simulink model "Drone_Model"  (R2019b)
settings: Solver=VariableStepAuto  StartTime=0.0  StopTime=6  RelTol=1e-3
values from neighbouring files (symbols this model uses):
  A = double(round(subs(J_x,   [states, inputs], [trim_state, trim_input])*1000)/1000)    [state_decoupling.m]
  Aaileron = A(5:8,5:8)    [state_decoupling.m]
  Aelevator = A(1:4,1:4)    [state_decoupling.m]
  Arudder = A(11:12,11:12)    [state_decoupling.m]
  Athrust = A(9:10,9:10)    [state_decoupling.m]
  B = B*MotorMix    [state_decoupling.m]
  Baileron = B(5:8,3)    [state_decoupling.m]
  Belevator = B(1:4,2)    [state_decoupling.m]
  Brudder = B(11:12,4)    [state_decoupling.m]
  Bthrust = B(9:10,1)    [state_decoupling.m]
  C = double(round(subs(J_y,   [states, inputs], [trim_state, trim_input])*1000)/1000)    [state_decoupling.m]
  C_P = 0.041    [state_decoupling.m]
  C_rollpitch = rho*prop_dia^4*prop_dist/sqrt(2)*[                 1  -1  -1   1 ;                 1   1  -1  -1 ;                 0   0   0   0 ; ]    [state_decoupling.m]
  C_T = [0.069075;4.95e-05]    [state_decoupling.m]
  C_yaw = rho*prop_dia^5/(2*pi)*[                 0   0   0   0 ;                 0   0   0   0 ;                -1   1  -1   1 ; ]    [state_decoupling.m]
  Caileron = [0 1 0 0; 0 0 0 1; 0 0 0 0]    [state_decoupling.m]
  Celevator = [0 1 0 0; 0 0 0 1; 0 0 0 0]    [state_decoupling.m]
  Crudder = [0 1]    [state_decoupling.m]
  Cthrust = [ 1 0; -1 0; 0 0]    [state_decoupling.m]
  D = D*MotorMix    [state_decoupling.m]
  Daileron = [0 ; 0 ; 0]    [state_decoupling.m]
  Delevator = [0 ; 0 ; 0]    [state_decoupling.m]
  Drudder = 0    [state_decoupling.m]
  Dthrust = [0 ; 0 ; D(4,1)]    [state_decoupling.m]
  g = [0;0;UAV_mass*9.81]    [state_decoupling.m]
  J = [      Jxx   0   0 ;       0   Jyy  0 ;       0    0  Jzz; ]    [state_decoupling.m]
  Jinv = inv(J)    [state_decoupling.m]
  MotorMix = [                 1  1  1 -1 ;                 1  1 -1  1 ;                 1 -1 -1 -1 ;                 1 -1  1  1 ; ]    [state_decoupling.m]
  Prop_H = 2*pi*Jprop*[               0  0  0  0 ;               0  0  0  0 ;               1 -1  1 -1 ; ]    [state_decoupling.m]
  Thrust_Sum = rho*prop_dia^4*[                 0   0   0   0 ;                 0   0   0   0 ;                -1  -1  -1  -1 ; ]    [state_decoupling.m]
  trim_input = [293,293,293,293]    [state_decoupling.m]
  trim_state = [0,0,0,0,0,0,0,0,0,0,0,0]    [state_decoupling.m]
  UAV_mass = 0.068    [state_decoupling.m]
undefined symbols (not defined in the file or in its folder): TEAR
libraries: simulink x8, vrlib x3, dspmtrx3 x1
settings Model: Creator=crbon  LastModifiedBy=Chris

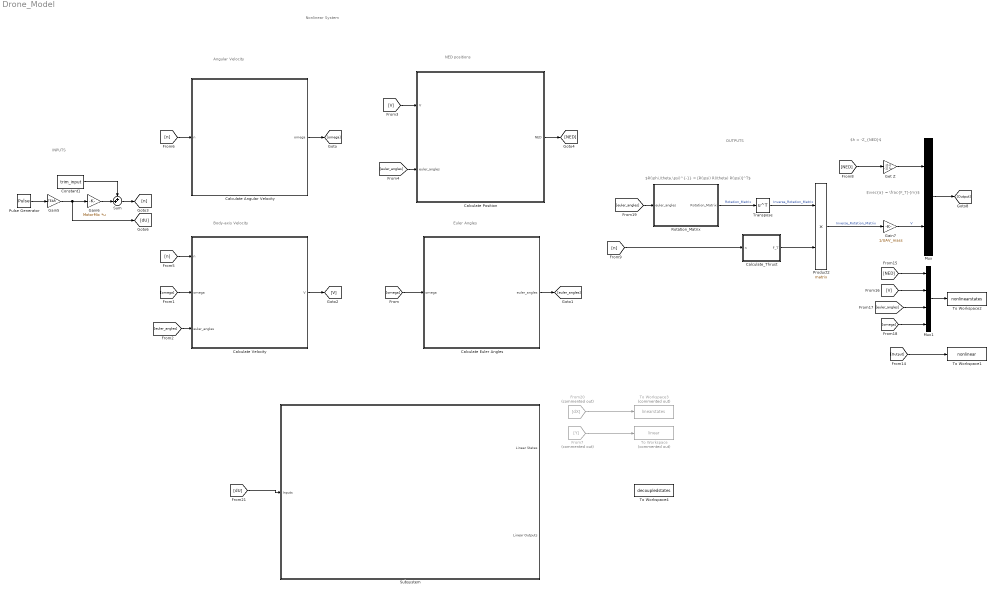
== system Drone_Model ==
  note: Nonlinear System
  note: Euler Angles
  note: NED positions
  note: $\vec{a} = \frac{F_T}{m}$
  note: $h = -Z_{NED}$
  note: $R(\phi,\theta,\psi)^{-1} = [R(\psi) R(\theta) R(\psi)]^T$
  note: OUTPUTS
  note: INPUTS
  note: Angular Velocity
  note: Body-axis Velocity
  Calculate Angular Velocity : Subsystem
  Calculate Euler Angles : Subsystem
  Calculate Position : Subsystem
  Calculate Velocity : Subsystem
  Calculate_Thrust : Subsystem
  Constant1 : Constant  Value=trim_input
  From20 : From  Commented=on  GotoTag=dX
  From7 : From  Commented=on  GotoTag=Y
  Gain5 : Gain  Gain=TEAR
      settings: AttributesFormatString=%<Gain>
  Gain6 : Gain  Gain=MotorMix  Multiplication=Matrix(K*u)
      settings: AttributesFormatString=%<Gain>
  Gain7 : Gain  Gain=1/UAV_mass
      settings: AttributesFormatString=%<Gain>
  Get Z : Gain  Gain=[0 0 -1]  Multiplication=Matrix(K*u)
  Mux : Mux  Inputs=2
  Mux1 : Mux
  Product2 : Product  Multiplication=Matrix(*)
  Pulse Generator : DiscretePulseGenerator  PulseType=Time based  Amplitude=0.05  Period=10  PulseWidth=40  PhaseDelay=1
  Rotation_Matrix : Subsystem
  Subsystem : Subsystem
  Sum : Sum  Inputs=++|
  To Workspace : ToWorkspace  Commented=on  VariableName=linear  SaveFormat=Timeseries  SampleTime=-1
  To Workspace1 : ToWorkspace  VariableName=nonlinear  SaveFormat=Timeseries  SampleTime=-1
  To Workspace2 : ToWorkspace  VariableName=nonlinearstates  SaveFormat=Timeseries  SampleTime=-1
  To Workspace3 : ToWorkspace  Commented=on  VariableName=linearstates  SaveFormat=Timeseries  SampleTime=-1
  To Workspace4 : ToWorkspace  VariableName=decoupledstates  SaveFormat=Timeseries  SampleTime=-1
  Transpose : Math  Operator=transpose  SignedPower=off  SaturateOnIntegerOverflow=on
  wires:
  [omega] -> Calculate Euler Angles/1(omega)
  Calculate Angular Velocity/1(omega) -> [omega]
  [omega] -> Calculate Velocity/2(omega)
  Calculate Euler Angles/1(euler_angles) -> [euler_angles]
  [euler_angles] -> Calculate Velocity/3(euler_angles)
  Calculate Velocity/1(V) -> [V]
  [V] -> Calculate Position/1("V ")
  [euler_angles] -> Calculate Position/2(euler_angles)
  [n] -> Calculate Velocity/1(n)
  [n] -> Calculate Angular Velocity/1(n)
  Calculate Position/1(NED) -> [NED]
  [NED] -> Get Z/1
  Get Z/1 -> Mux/1
  [n] -> Calculate_Thrust/1(n)
  Calculate_Thrust/1(F_T) -> Product2/2
  Gain7/1 -> Mux/2  "V"
  Mux/1 -> [Output]
  From7/1 -> To Workspace/1
  [Output] -> To Workspace1/1
  Constant1/1 -> Sum/1
  [NED] -> Mux1/1
  [V] -> Mux1/2
  [euler_angles] -> Mux1/3
  [omega] -> Mux1/4
  Mux1/1 -> To Workspace2/1
  Pulse Generator/1 -> Gain5/1
  Product2/1 -> Gain7/1  "Inverse_Rotation_Matrix"
  Rotation_Matrix/1(Rotation_Matrix) -> Transpose/1  "Rotation_Matrix"
  [euler_angles] -> Rotation_Matrix/1("euler_angles ")
  Transpose/1 -> Product2/1  "Inverse_Rotation_Matrix"
  From20/1 -> To Workspace3/1
  Gain5/1 -> Gain6/1, [dU]
  Sum/1 -> [n]
  Gain6/1 -> Sum/2
  [dU] -> Subsystem/1("Inputs ")

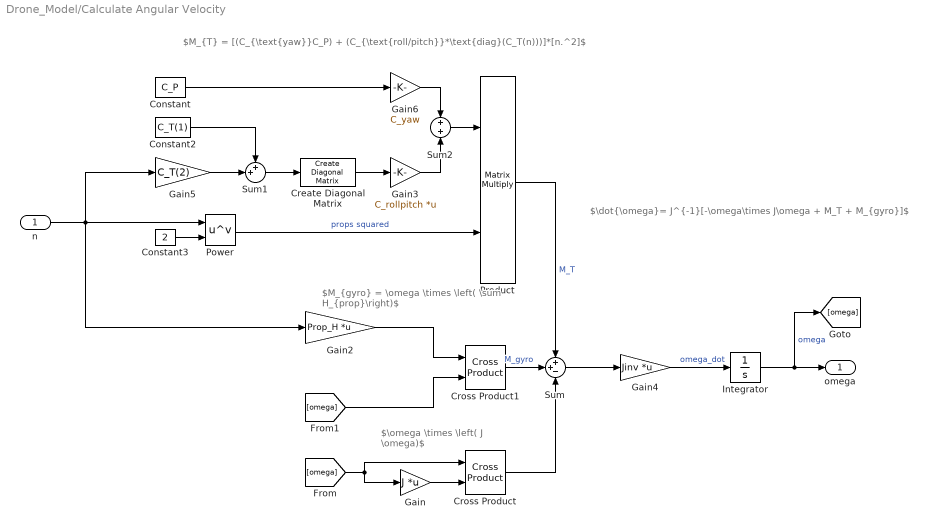
== system Drone_Model/Calculate Angular Velocity ==
  note: $M_{gyro} = \omega \times \left( \sum H_{prop}\right)$
  note: $\dot{\omega}= J^{-1}[-\omega\times J\omega + M_T + M_{gyro}]$
  note: $\omega \times \left( J \omega)$
  note: $M_{T} = [(C_{\text{yaw}}C_P) + (C_{\text{roll/pitch}}*\text{diag}(C_T(n)))]*[n.^2]$
  n : Inport
  Constant : Constant  Value=C_P
  Constant2 : Constant  Value=C_T(1)
  Constant3 : Constant  Value=2
  Create Diagonal Matrix : dspmtrx3/Create Diagonal Matrix
      settings: SourceProductName=DSP System Toolbox  SourceProductBaseCode=DS
  Cross Product : vrlib/Utilities/Cross Product
      settings: SourceProductName=Simulink
  Cross Product1 : vrlib/Utilities/Cross Product
      settings: SourceProductName=Simulink
  Gain : Gain  Gain=J  Multiplication=Matrix(K*u)
  Gain2 : Gain  Gain=Prop_H  Multiplication=Matrix(K*u)
  Gain3 : Gain  Gain=C_rollpitch  Multiplication=Matrix(K*u)
      settings: AttributesFormatString=%<Gain>
  Gain4 : Gain  Gain=Jinv  Multiplication=Matrix(K*u)
      settings: AttributesFormatString=%<Gain>
  Gain5 : Gain  Gain=C_T(2)
  Gain6 : Gain  Gain=C_yaw
      settings: AttributesFormatString=%<Gain>
  Integrator : Integrator  InitialCondition=[0;0;0]
  Power : Math  Operator=pow  SignedPower=off  SaturateOnIntegerOverflow=on
  Product : Product  Multiplication=Matrix(*)
  Sum : Sum  Inputs=++-
  Sum1 : Sum  Inputs=++|
  Sum2 : Sum  Inputs=+|+
  omega : Outport
  wires:
  Sum/1 -> Gain4/1
  [omega] -> Gain/1, Cross Product/1
  Cross Product/1 -> Sum/3
  [omega] -> Cross Product1/2
  Gain2/1 -> Cross Product1/1
  Cross Product1/1 -> Sum/2  "M_gyro"
  Gain4/1 -> Integrator/1  "omega_dot"
  Gain/1 -> Cross Product/2
  Integrator/1 -> [omega], omega/1  "omega"
  Product/1 -> Sum/1  "M_T"
  Create Diagonal Matrix/1 -> Gain3/1
  Sum2/1 -> Product/1
  Sum1/1 -> Create Diagonal Matrix/1
  Constant/1 -> Gain6/1
  Power/1 -> Product/2  "props squared"
  Gain6/1 -> Sum2/1
  Gain5/1 -> Sum1/2
  Gain3/1 -> Sum2/2
  n/1 -> Gain2/1, Power/1, Gain5/1
  Constant2/1 -> Sum1/1
  Constant3/1 -> Power/2

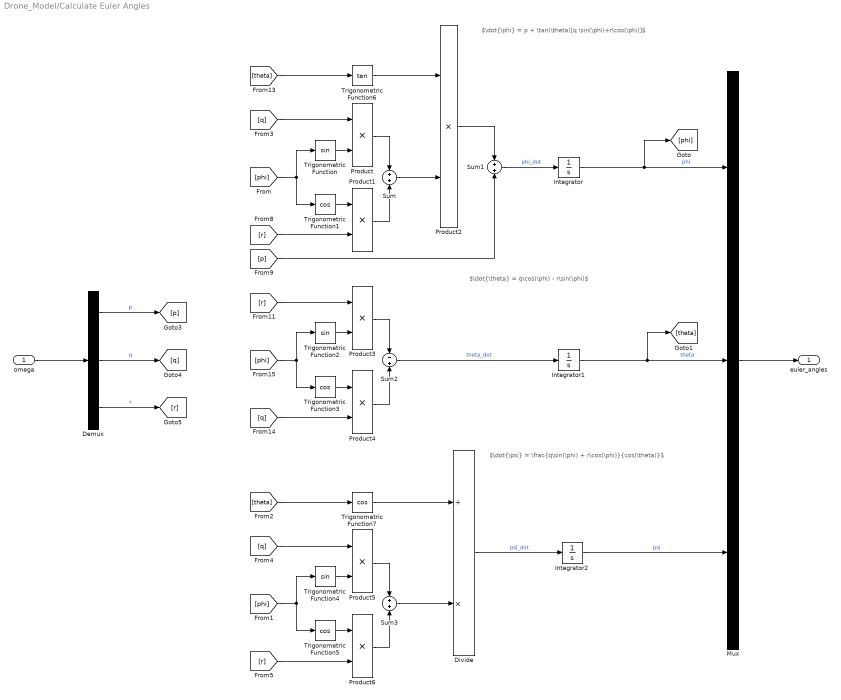
== system Drone_Model/Calculate Euler Angles ==
  note: $\dot{\phi} = p + \tan(\theta)[q \sin(\phi)+r\cos(\phi)]$
  note: $\dot{\theta} = q\cos(\phi) - r\sin(\phi)$
  note: $\dot{\psi} = \frac{q\sin(\phi) + r\cos(\phi)}{cos(\theta)}$
  omega : Inport
  Demux : Demux  Outputs=3
  Divide : Product  Inputs=/*
  Integrator : Integrator
  Integrator1 : Integrator
  Integrator2 : Integrator
  Mux : Mux  Inputs=3
  Product{,1..6} (7 alike) : Product
  Sum : Sum  Inputs=+|+
  Sum1 : Sum  Inputs=+|+
  Sum2 : Sum  Inputs=-|+
  Sum3 : Sum  Inputs=+|+
  Trigonometric Function : Trigonometry
  Trigonometric Function{1,3,5,7} (4 alike) : Trigonometry  Operator=cos
  Trigonometric Function2 : Trigonometry
  Trigonometric Function4 : Trigonometry
  Trigonometric Function6 : Trigonometry  Operator=tan
  euler_angles : Outport
  wires:
  Trigonometric Function7/1 -> Divide/1
  Product1/1 -> Sum/2
  Product6/1 -> Sum3/2
  Trigonometric Function/1 -> Product/2
  Product5/1 -> Sum3/1
  [theta] -> Trigonometric Function7/1
  Trigonometric Function6/1 -> Product2/1
  [r] -> Product6/2
  [theta] -> Trigonometric Function6/1
  Integrator1/1 -> [theta], Mux/2  "theta"
  Trigonometric Function4/1 -> Product5/2
  [q] -> Product4/2
  Demux/3 -> [r]  "r"
  Divide/1 -> Integrator2/1  "psi_dot"
  Integrator2/1 -> Mux/3  "psi"
  [q] -> Product5/1
  Product4/1 -> Sum2/2
  [q] -> Product/1
  [phi] -> Trigonometric Function4/1, Trigonometric Function5/1
  Sum2/1 -> Integrator1/1  "theta_dot"
  Trigonometric Function5/1 -> Product6/1
  Trigonometric Function3/1 -> Product4/1
  [r] -> Product3/1
  Integrator/1 -> [phi], Mux/1  "phi"
  Sum3/1 -> Divide/2
  Product3/1 -> Sum2/1
  [phi] -> Trigonometric Function2/1, Trigonometric Function3/1
  Demux/1 -> [p]  "p"
  Product2/1 -> Sum1/1
  [r] -> Product1/2
  Trigonometric Function1/1 -> Product1/1
  [phi] -> Trigonometric Function1/1, Trigonometric Function/1
  omega/1 -> Demux/1
  Product/1 -> Sum/1
  Demux/2 -> [q]  "q"
  Sum/1 -> Product2/2
  Mux/1 -> euler_angles/1
  Sum1/1 -> Integrator/1  "phi_dot"
  [p] -> Sum1/2
  Trigonometric Function2/1 -> Product3/2

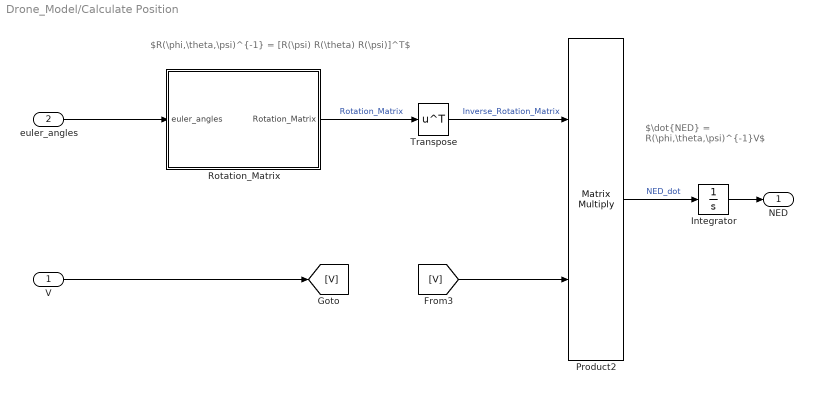
== system Drone_Model/Calculate Position ==
  note: $R(\phi,\theta,\psi)^{-1} = [R(\psi) R(\theta) R(\psi)]^T$
  note: $\dot{NED} = R(\phi,\theta,\psi)^{-1}V$
  "V " : Inport
  euler_angles : Inport  Port=2
  Integrator : Integrator  InitialCondition=[0;0;0]
  Product2 : Product  Multiplication=Matrix(*)
  Rotation_Matrix : Subsystem
  Transpose : Math  Operator=transpose  SignedPower=off  SaturateOnIntegerOverflow=on
  NED : Outport
  wires:
  Product2/1 -> Integrator/1  "NED_dot"
  "V "/1 -> [V]
  Rotation_Matrix/1(Rotation_Matrix) -> Transpose/1  "Rotation_Matrix"
  Transpose/1 -> Product2/1  "Inverse_Rotation_Matrix"
  [V] -> Product2/2
  euler_angles/1 -> Rotation_Matrix/1("euler_angles ")
  Integrator/1 -> NED/1

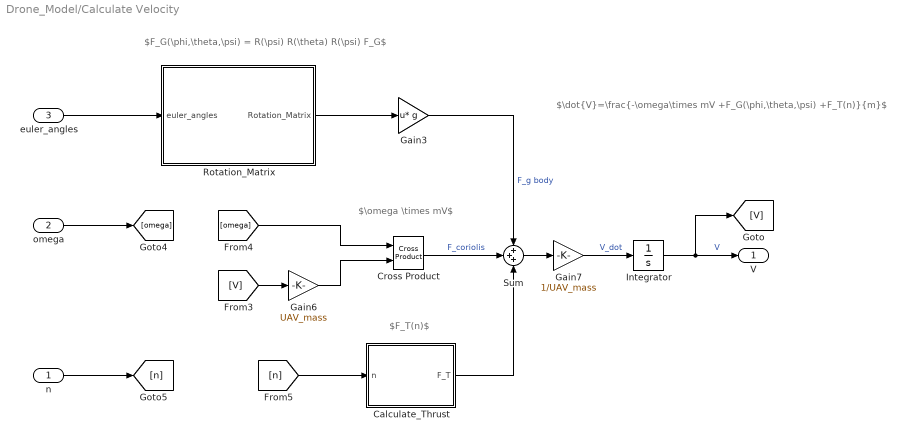
== system Drone_Model/Calculate Velocity ==
  note: $F_G(\phi,\theta,\psi) = R(\psi) R(\theta) R(\psi) F_G$
  note: $\dot{V}=\frac{-\omega\times mV +F_G(\phi,\theta,\psi) +F_T(n)}{m}$
  note: $\omega \times mV$
  note: $F_T(n)$
  n : Inport
  omega : Inport  Port=2
  euler_angles : Inport  Port=3
  Calculate_Thrust : Subsystem
  Cross Product : vrlib/Utilities/Cross Product
      settings: SourceProductName=Simulink
  Gain3 : Gain  Gain=g  Multiplication=Matrix(u*K)
      settings: AttributesFormatString=%<Gain>
  Gain6 : Gain  Gain=UAV_mass
      settings: AttributesFormatString=%<Gain>
  Gain7 : Gain  Gain=1/UAV_mass
      settings: AttributesFormatString=%<Gain>
  Integrator : Integrator  InitialCondition=[0;0;0]
  Rotation_Matrix : Subsystem
  Sum : Sum  Inputs=+++
  V : Outport
  wires:
  [V] -> Gain6/1
  [omega] -> Cross Product/1
  Cross Product/1 -> Sum/2  "F_coriolis"
  Gain3/1 -> Sum/1  "F_g body"
  Gain6/1 -> Cross Product/2
  Sum/1 -> Gain7/1
  Integrator/1 -> V/1, [V]  "V"
  omega/1 -> [omega]
  n/1 -> [n]
  Rotation_Matrix/1(Rotation_Matrix) -> Gain3/1
  euler_angles/1 -> Rotation_Matrix/1("euler_angles ")
  [n] -> Calculate_Thrust/1(n)
  Gain7/1 -> Integrator/1  "V_dot"
  Calculate_Thrust/1(F_T) -> Sum/3

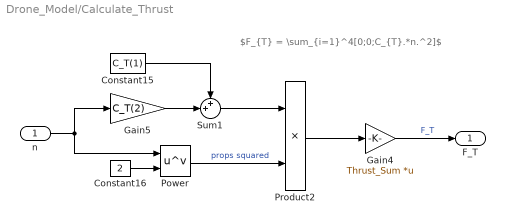
== system Drone_Model/Calculate_Thrust ==
  note: $F_{T} = \sum_{i=1}^4[0;0;C_{T}.*n.^2]$
  n : Inport
  Constant15 : Constant  Value=C_T(1)
  Constant16 : Constant  Value=2
  Gain4 : Gain  Gain=Thrust_Sum  Multiplication=Matrix(K*u)
      settings: AttributesFormatString=%<Gain>
  Gain5 : Gain  Gain=C_T(2)
  Power : Math  Operator=pow  SignedPower=off  SaturateOnIntegerOverflow=on
  Product2 : Product
  Sum1 : Sum  Inputs=++|
  F_T : Outport
  wires:
  Constant15/1 -> Sum1/1
  Gain4/1 -> F_T/1  "F_T"
  n/1 -> Power/1, Gain5/1
  Power/1 -> Product2/2  "props squared"
  Gain5/1 -> Sum1/2
  Sum1/1 -> Product2/1
  Product2/1 -> Gain4/1
  Constant16/1 -> Power/2

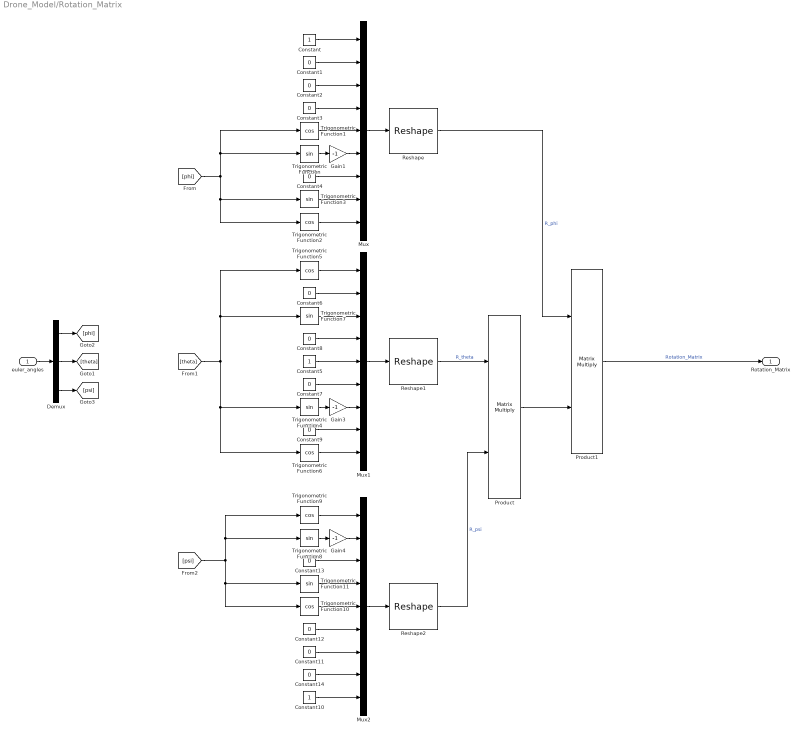
== system Drone_Model/Rotation_Matrix ==
  "euler_angles " : Inport
  Constant : Constant
  Constant{1..4,6..9,11..14} (12 alike) : Constant  Value=0
  Constant10 : Constant
  Constant5 : Constant
  Demux : Demux  Outputs=3
  Gain1 : Gain  Gain=-1
  Gain3 : Gain  Gain=-1
  Gain4 : Gain  Gain=-1
  Mux : Mux  Inputs=9
  Mux1 : Mux  Inputs=9
  Mux2 : Mux  Inputs=9
  Product : Product  Multiplication=Matrix(*)
  Product1 : Product  Multiplication=Matrix(*)
  Reshape : Reshape  OutputDimensionality=Customize  OutputDimensions=[3,3]
  Reshape1 : Reshape  OutputDimensionality=Customize  OutputDimensions=[3,3]
  Reshape2 : Reshape  OutputDimensionality=Customize  OutputDimensions=[3,3]
  Trigonometric Function{,3..4,7..8,11} (6 alike) : Trigonometry
  Trigonometric Function{1..2,5..6,9..10} (6 alike) : Trigonometry  Operator=cos
  Rotation_Matrix : Outport
  wires:
  Constant9/1 -> Mux1/8
  Constant11/1 -> Mux2/7
  Trigonometric Function1/1 -> Mux/5
  Trigonometric Function3/1 -> Mux/8
  Constant5/1 -> Mux1/5
  Trigonometric Function7/1 -> Mux1/3
  Reshape/1 -> Product1/1  "R_phi"
  Mux1/1 -> Reshape1/1
  Trigonometric Function8/1 -> Gain4/1
  Constant7/1 -> Mux1/6
  Trigonometric Function2/1 -> Mux/9
  [phi] -> Trigonometric Function2/1, Trigonometric Function3/1, Trigonometric Function1/1, Trigonometric Function/1
  Trigonometric Function6/1 -> Mux1/9
  Constant12/1 -> Mux2/6
  Trigonometric Function4/1 -> Gain3/1
  [theta] -> Trigonometric Function7/1, Trigonometric Function5/1, Trigonometric Function4/1, Trigonometric Function6/1
  Reshape2/1 -> Product/2  "R_psi"
  Trigonometric Function/1 -> Gain1/1
  Product/1 -> Product1/2
  Trigonometric Function5/1 -> Mux1/1
  Trigonometric Function9/1 -> Mux2/1
  Mux/1 -> Reshape/1
  Constant/1 -> Mux/1
  Constant3/1 -> Mux/4
  Constant6/1 -> Mux1/2
  Mux2/1 -> Reshape2/1
  Constant2/1 -> Mux/3
  Constant1/1 -> Mux/2
  [psi] -> Trigonometric Function11/1, Trigonometric Function10/1, Trigonometric Function9/1, Trigonometric Function8/1
  Constant8/1 -> Mux1/4
  Constant4/1 -> Mux/7
  Constant13/1 -> Mux2/3
  Trigonometric Function11/1 -> Mux2/4
  Constant10/1 -> Mux2/9
  Reshape1/1 -> Product/1  "R_theta"
  Constant14/1 -> Mux2/8
  Trigonometric Function10/1 -> Mux2/5
  Product1/1 -> Rotation_Matrix/1  "Rotation_Matrix"
  Demux/3 -> [psi]
  Demux/2 -> [theta]
  "euler_angles "/1 -> Demux/1
  Demux/1 -> [phi]
  Gain3/1 -> Mux1/7
  Gain1/1 -> Mux/6
  Gain4/1 -> Mux2/2

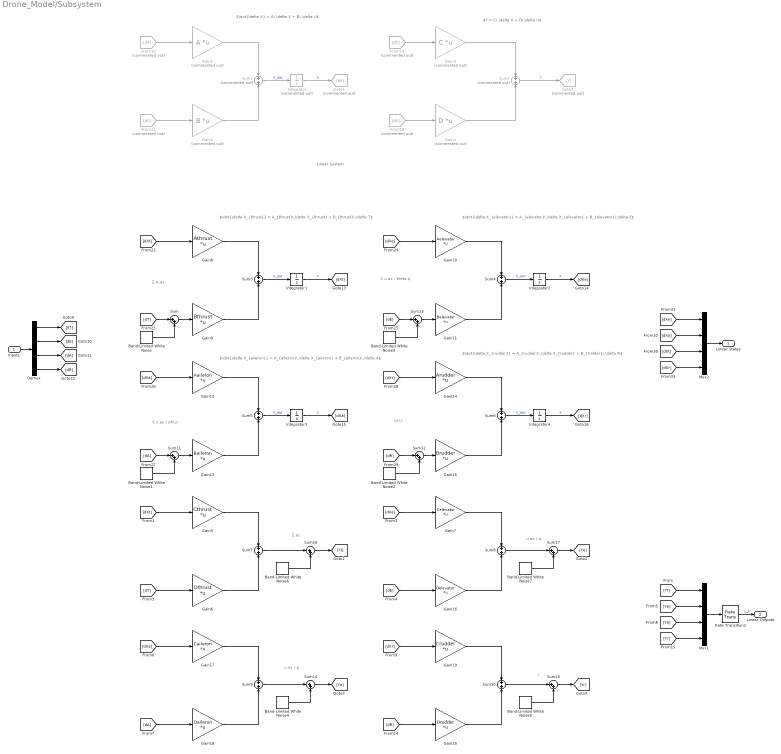
== system Drone_Model/Subsystem ==
  note: psi,r
  note: Y,v,ay / phi,p
  note: X,u,ax / theta,q
  note: Z,w,az
  note: Linear System
  note: $\dot{\delta X} = A\,\delta X + B\,\delta U$
  note: $Y = C\,\delta X + D\,\delta U$
  note: $\dot{\delta X_{thrust}} = A_{thrust}\,\delta X_{thrust} + B_{thrust}\,\delta T$
  note: $\dot{\delta X_{elevator}} = A_{elevator}\,\delta X_{elevator} + B_{elevator}\,\delta E$
  note: $\dot{\delta X_{aileron}} = A_{aileron}\,\delta X_{aileron} + B_{aileron}\,\delta A$
  note: $\dot{\delta X_{rudder}} = A_{rudder}\,\delta X_{rudder} + B_{rudder}\,\delta R$
  note: Z,az
  note: u,ax / q
  note: v,ay / p
  note: r
  "Inputs " : Inport
  Band-Limited White Noise : simulink/Sources/Band-Limited White Noise  Cov=0.1  Ts=0.1  seed=45
  Band-Limited White Noise{1,4..7} (5 alike) : simulink/Sources/Band-Limited White Noise  Cov=0.1  Ts=0.1  seed=20
  Band-Limited White Noise2 : simulink/Sources/Band-Limited White Noise  Cov=0.1  Ts=0.1  seed=[10]
  Band-Limited White Noise3 : simulink/Sources/Band-Limited White Noise  Cov=0.1  Ts=0.1  seed=435345
  Demux : Demux
  From10 : From  Commented=on  GotoTag=dX
  From11 : From  Commented=on  GotoTag=dU
  From12 : From  Commented=on  GotoTag=dX
  From13 : From  Commented=on  GotoTag=dU
  Gain1 : Gain  Commented=on  Gain=A  Multiplication=Matrix(K*u)
  Gain10 : Gain  Gain=Aelevator  Multiplication=Matrix(K*u)
  Gain11 : Gain  Gain=Belevator  Multiplication=Matrix(K*u)
  Gain12 : Gain  Gain=Aaileron  Multiplication=Matrix(K*u)
  Gain13 : Gain  Gain=Baileron  Multiplication=Matrix(K*u)
  Gain14 : Gain  Gain=Arudder  Multiplication=Matrix(K*u)
  Gain15 : Gain  Gain=Brudder  Multiplication=Matrix(K*u)
  Gain16 : Gain  Gain=Delevator  Multiplication=Matrix(K*u)
  Gain17 : Gain  Gain=Caileron  Multiplication=Matrix(K*u)
  Gain18 : Gain  Gain=Daileron  Multiplication=Matrix(K*u)
  Gain19 : Gain  Gain=Crudder  Multiplication=Matrix(K*u)
  Gain2 : Gain  Commented=on  Gain=B  Multiplication=Matrix(K*u)
  Gain20 : Gain  Gain=Drudder  Multiplication=Matrix(K*u)
  Gain3 : Gain  Commented=on  Gain=C  Multiplication=Matrix(K*u)
  Gain4 : Gain  Commented=on  Gain=D  Multiplication=Matrix(K*u)
  Gain5 : Gain  Gain=Cthrust  Multiplication=Matrix(K*u)
  Gain6 : Gain  Gain=Dthrust  Multiplication=Matrix(K*u)
  Gain7 : Gain  Gain=Celevator  Multiplication=Matrix(K*u)
  Gain8 : Gain  Gain=Athrust  Multiplication=Matrix(K*u)
  Gain9 : Gain  Gain=Bthrust  Multiplication=Matrix(K*u)
  Goto5 : Goto  Commented=on  GotoTag=dX
  Goto7 : Goto  Commented=on  GotoTag=Y
  Integrator : Integrator  Commented=on  InitialCondition=trim_state
  Integrator1 : Integrator  InitialCondition=trim_state(9:10)
  Integrator2 : Integrator  InitialCondition=trim_state(1:4)
  Integrator3 : Integrator  InitialCondition=trim_state(5:8)
  Integrator4 : Integrator  InitialCondition=trim_state(11:12)
  Mux1 : Mux
  Mux2 : Mux
  Rate Transition2 : RateTransition  OutPortSampleTime=0.005
  Sum{,11..17} (8 alike) : Sum  Inputs=|++
  Sum1 : Sum  Commented=on  Inputs=+|+
  Sum{3..10} (8 alike) : Sum  Inputs=+|+
  Sum2 : Sum  Commented=on  Inputs=+|+
  Linear States : Outport
  Linear Outputs : Outport  Port=2
  wires:
  Gain14/1 -> Sum6/1
  From11/1 -> Gain2/1
  [dXe] -> Gain10/1
  Gain10/1 -> Sum4/1
  Gain2/1 -> Sum1/2
  Gain15/1 -> Sum6/2
  Gain1/1 -> Sum1/1
  Sum5/1 -> Integrator3/1  "X_dot"
  Gain3/1 -> Sum2/1
  Integrator1/1 -> [dXt]  "X"
  From10/1 -> Gain1/1
  Sum1/1 -> Integrator/1  "X_dot"
  Sum2/1 -> Goto7/1  "Y"
  Integrator3/1 -> [dXa]  "X"
  Gain8/1 -> Sum3/1
  [dXt] -> Gain8/1
  Sum3/1 -> Integrator1/1  "X_dot"
  Integrator4/1 -> [dXr]  "X"
  Sum4/1 -> Integrator2/1  "X_dot"
  Gain13/1 -> Sum5/2
  [dXa] -> Gain12/1
  [dXr] -> Gain14/1
  Gain9/1 -> Sum3/2
  Sum6/1 -> Integrator4/1  "X_dot"
  From13/1 -> Gain4/1
  Gain11/1 -> Sum4/2
  Integrator/1 -> Goto5/1  "X"
  Gain4/1 -> Sum2/2
  Gain12/1 -> Sum5/1
  Integrator2/1 -> [dXe]  "X"
  From12/1 -> Gain3/1
  "Inputs "/1 -> Demux/1
  Demux/3 -> [dA]
  Demux/2 -> [dE]
  Demux/1 -> [dT]
  Demux/4 -> [dR]
  [dXt] -> Mux2/3
  [dXr] -> Mux2/4
  Mux2/1 -> Linear States/1
  [dXe] -> Mux2/1
  [dXa] -> Mux2/2
  Gain6/1 -> Sum7/2
  [dT] -> Gain6/1
  [dXt] -> Gain5/1
  Gain5/1 -> Sum7/1
  Gain16/1 -> Sum8/2
  [dE] -> Gain16/1
  Gain7/1 -> Sum8/1
  [dXe] -> Gain7/1
  [dA] -> Gain18/1
  Gain17/1 -> Sum9/1
  [dXa] -> Gain17/1
  Gain18/1 -> Sum9/2
  [dXr] -> Gain19/1
  [dR] -> Gain20/1
  Gain20/1 -> Sum10/2
  Gain19/1 -> Sum10/1
  [Ye] -> Mux1/2
  [Yt] -> Mux1/1
  Mux1/1 -> Rate Transition2/1
  [Yr] -> Mux1/4
  [Ya] -> Mux1/3
  Band-Limited White Noise/1 -> Sum/2
  [dT] -> Sum/1
  Sum/1 -> Gain9/1
  Sum11/1 -> Gain13/1
  [dA] -> Sum11/1
  Band-Limited White Noise1/1 -> Sum11/2
  Band-Limited White Noise2/1 -> Sum12/2
  [dR] -> Sum12/1
  Sum12/1 -> Gain15/1
  Sum13/1 -> Gain11/1
  [dE] -> Sum13/1
  Band-Limited White Noise3/1 -> Sum13/2
  Band-Limited White Noise4/1 -> Sum14/2
  Sum9/1 -> Sum14/1
  Sum14/1 -> [Ya]
  Sum15/1 -> [Yr]
  Sum10/1 -> Sum15/1
  Band-Limited White Noise5/1 -> Sum15/2
  Band-Limited White Noise6/1 -> Sum16/2
  Sum7/1 -> Sum16/1
  Sum16/1 -> [Yt]
  Band-Limited White Noise7/1 -> Sum17/2
  Sum8/1 -> Sum17/1
  Sum17/1 -> [Ye]
  Rate Transition2/1 -> Linear Outputs/1  "y_k"

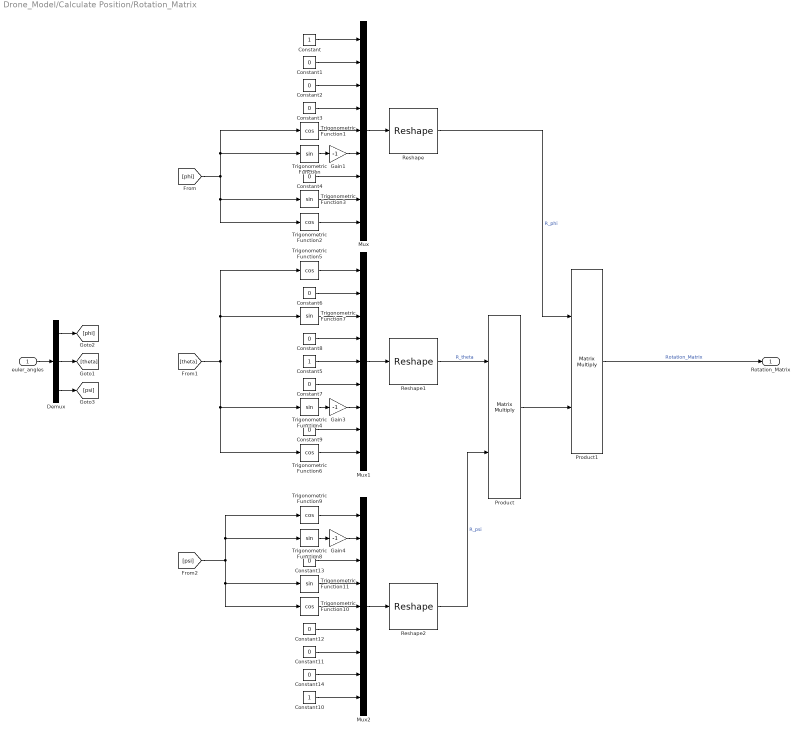
== system Drone_Model/Calculate Position/Rotation_Matrix ==
  "euler_angles " : Inport
  Constant : Constant
  Constant{1..4,6..9,11..14} (12 alike) : Constant  Value=0
  Constant10 : Constant
  Constant5 : Constant
  Demux : Demux  Outputs=3
  Gain1 : Gain  Gain=-1
  Gain3 : Gain  Gain=-1
  Gain4 : Gain  Gain=-1
  Mux : Mux  Inputs=9
  Mux1 : Mux  Inputs=9
  Mux2 : Mux  Inputs=9
  Product : Product  Multiplication=Matrix(*)
  Product1 : Product  Multiplication=Matrix(*)
  Reshape : Reshape  OutputDimensionality=Customize  OutputDimensions=[3,3]
  Reshape1 : Reshape  OutputDimensionality=Customize  OutputDimensions=[3,3]
  Reshape2 : Reshape  OutputDimensionality=Customize  OutputDimensions=[3,3]
  Trigonometric Function{,3..4,7..8,11} (6 alike) : Trigonometry
  Trigonometric Function{1..2,5..6,9..10} (6 alike) : Trigonometry  Operator=cos
  Rotation_Matrix : Outport
  wires:
  Constant9/1 -> Mux1/8
  Constant11/1 -> Mux2/7
  Trigonometric Function1/1 -> Mux/5
  Trigonometric Function3/1 -> Mux/8
  Constant5/1 -> Mux1/5
  Trigonometric Function7/1 -> Mux1/3
  Reshape/1 -> Product1/1  "R_phi"
  Mux1/1 -> Reshape1/1
  Trigonometric Function8/1 -> Gain4/1
  Constant7/1 -> Mux1/6
  Trigonometric Function2/1 -> Mux/9
  [phi] -> Trigonometric Function2/1, Trigonometric Function3/1, Trigonometric Function1/1, Trigonometric Function/1
  Trigonometric Function6/1 -> Mux1/9
  Constant12/1 -> Mux2/6
  Trigonometric Function4/1 -> Gain3/1
  [theta] -> Trigonometric Function7/1, Trigonometric Function5/1, Trigonometric Function4/1, Trigonometric Function6/1
  Reshape2/1 -> Product/2  "R_psi"
  Trigonometric Function/1 -> Gain1/1
  Product/1 -> Product1/2
  Trigonometric Function5/1 -> Mux1/1
  Trigonometric Function9/1 -> Mux2/1
  Mux/1 -> Reshape/1
  Constant/1 -> Mux/1
  Constant3/1 -> Mux/4
  Constant6/1 -> Mux1/2
  Mux2/1 -> Reshape2/1
  Constant2/1 -> Mux/3
  Constant1/1 -> Mux/2
  [psi] -> Trigonometric Function11/1, Trigonometric Function10/1, Trigonometric Function9/1, Trigonometric Function8/1
  Constant8/1 -> Mux1/4
  Constant4/1 -> Mux/7
  Constant13/1 -> Mux2/3
  Trigonometric Function11/1 -> Mux2/4
  Constant10/1 -> Mux2/9
  Reshape1/1 -> Product/1  "R_theta"
  Constant14/1 -> Mux2/8
  Trigonometric Function10/1 -> Mux2/5
  Product1/1 -> Rotation_Matrix/1  "Rotation_Matrix"
  Demux/3 -> [psi]
  Demux/2 -> [theta]
  "euler_angles "/1 -> Demux/1
  Demux/1 -> [phi]
  Gain3/1 -> Mux1/7
  Gain1/1 -> Mux/6
  Gain4/1 -> Mux2/2

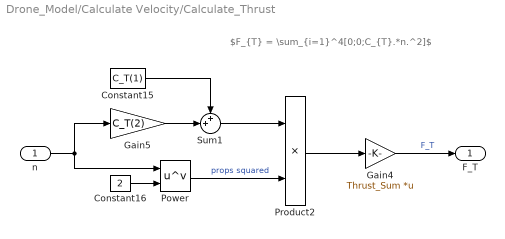
== system Drone_Model/Calculate Velocity/Calculate_Thrust ==
  note: $F_{T} = \sum_{i=1}^4[0;0;C_{T}.*n.^2]$
  n : Inport
  Constant15 : Constant  Value=C_T(1)
  Constant16 : Constant  Value=2
  Gain4 : Gain  Gain=Thrust_Sum  Multiplication=Matrix(K*u)
      settings: AttributesFormatString=%<Gain>
  Gain5 : Gain  Gain=C_T(2)
  Power : Math  Operator=pow  SignedPower=off  SaturateOnIntegerOverflow=on
  Product2 : Product
  Sum1 : Sum  Inputs=++|
  F_T : Outport
  wires:
  Constant15/1 -> Sum1/1
  Gain4/1 -> F_T/1  "F_T"
  n/1 -> Power/1, Gain5/1
  Power/1 -> Product2/2  "props squared"
  Gain5/1 -> Sum1/2
  Sum1/1 -> Product2/1
  Product2/1 -> Gain4/1
  Constant16/1 -> Power/2

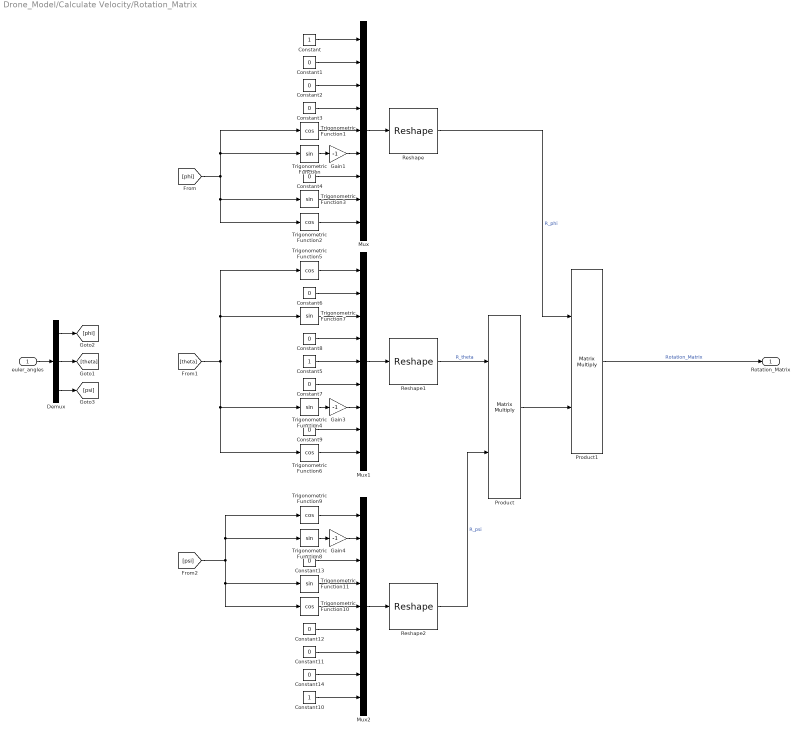
== system Drone_Model/Calculate Velocity/Rotation_Matrix ==
  "euler_angles " : Inport
  Constant : Constant
  Constant{1..4,6..9,11..14} (12 alike) : Constant  Value=0
  Constant10 : Constant
  Constant5 : Constant
  Demux : Demux  Outputs=3
  Gain1 : Gain  Gain=-1
  Gain3 : Gain  Gain=-1
  Gain4 : Gain  Gain=-1
  Mux : Mux  Inputs=9
  Mux1 : Mux  Inputs=9
  Mux2 : Mux  Inputs=9
  Product : Product  Multiplication=Matrix(*)
  Product1 : Product  Multiplication=Matrix(*)
  Reshape : Reshape  OutputDimensionality=Customize  OutputDimensions=[3,3]
  Reshape1 : Reshape  OutputDimensionality=Customize  OutputDimensions=[3,3]
  Reshape2 : Reshape  OutputDimensionality=Customize  OutputDimensions=[3,3]
  Trigonometric Function{,3..4,7..8,11} (6 alike) : Trigonometry
  Trigonometric Function{1..2,5..6,9..10} (6 alike) : Trigonometry  Operator=cos
  Rotation_Matrix : Outport
  wires:
  Constant9/1 -> Mux1/8
  Constant11/1 -> Mux2/7
  Trigonometric Function1/1 -> Mux/5
  Trigonometric Function3/1 -> Mux/8
  Constant5/1 -> Mux1/5
  Trigonometric Function7/1 -> Mux1/3
  Reshape/1 -> Product1/1  "R_phi"
  Mux1/1 -> Reshape1/1
  Trigonometric Function8/1 -> Gain4/1
  Constant7/1 -> Mux1/6
  Trigonometric Function2/1 -> Mux/9
  [phi] -> Trigonometric Function2/1, Trigonometric Function3/1, Trigonometric Function1/1, Trigonometric Function/1
  Trigonometric Function6/1 -> Mux1/9
  Constant12/1 -> Mux2/6
  Trigonometric Function4/1 -> Gain3/1
  [theta] -> Trigonometric Function7/1, Trigonometric Function5/1, Trigonometric Function4/1, Trigonometric Function6/1
  Reshape2/1 -> Product/2  "R_psi"
  Trigonometric Function/1 -> Gain1/1
  Product/1 -> Product1/2
  Trigonometric Function5/1 -> Mux1/1
  Trigonometric Function9/1 -> Mux2/1
  Mux/1 -> Reshape/1
  Constant/1 -> Mux/1
  Constant3/1 -> Mux/4
  Constant6/1 -> Mux1/2
  Mux2/1 -> Reshape2/1
  Constant2/1 -> Mux/3
  Constant1/1 -> Mux/2
  [psi] -> Trigonometric Function11/1, Trigonometric Function10/1, Trigonometric Function9/1, Trigonometric Function8/1
  Constant8/1 -> Mux1/4
  Constant4/1 -> Mux/7
  Constant13/1 -> Mux2/3
  Trigonometric Function11/1 -> Mux2/4
  Constant10/1 -> Mux2/9
  Reshape1/1 -> Product/1  "R_theta"
  Constant14/1 -> Mux2/8
  Trigonometric Function10/1 -> Mux2/5
  Product1/1 -> Rotation_Matrix/1  "Rotation_Matrix"
  Demux/3 -> [psi]
  Demux/2 -> [theta]
  "euler_angles "/1 -> Demux/1
  Demux/1 -> [phi]
  Gain3/1 -> Mux1/7
  Gain1/1 -> Mux/6
  Gain4/1 -> Mux2/2
